simulink model "MPC_point_3"  (R2022a)
settings: Solver=VariableStepAuto  StartTime=0.0  StopTime=T_sim  RelTol=1e-3
values from neighbouring files (symbols this model uses):
  C = [0       1      0  0 ... (first row only)    [main.m]
  C_states = eye(length(A))    [main.m]
  D_states = zeros(length(B), 1)    [main.m]
  N1 = 15    [main.m]
  N2 = 15    [main.m]
  N3 = 100    [main.m]
  N4 = 5    [main.m]
  Q1 = Q_d    [main.m]
  Q2 = Q_d    [main.m]
  Q3 = Q_d    [main.m]
  Q4 = Q_d    [main.m]
  R1 = R_d    (= 10000)    [main.m]
  R2 = R_d    (= 10000)    [main.m]
  R3 = R_d    (= 10000)    [main.m]
  R4 = R_d    (= 10000)    [main.m]
  S1 = Q_d    [main.m]
  S2 = 100 * Q_d    [main.m]
  S3 = Q_d    [main.m]
  S4 = P_d    [main.m]
  sysd = c2d(sys,T_sampling)    [main.m]
  T_sampling = 2*pi/omega_sampling    [main.m]
  u_max = deg2rad(15)    [main.m]
  u_min = deg2rad(-15)    [main.m]
  x0 = [deg2rad(0) deg2rad(15) 0 -300]    [main.m]
  x_ref = [0 0 0 0]    [main.m]
undefined symbols (not defined in the file or in its folder): Klqr_d, mpc_point_3
settings Model: Creator=PaoloA  LastModifiedBy=g_mor
settings DebuggingCC: UnconnectedInputMsg=warning  UnconnectedOutputMsg=warning  UnconnectedLineMsg=warning
settings RTWCC: DLArmComputeVersion=19.05

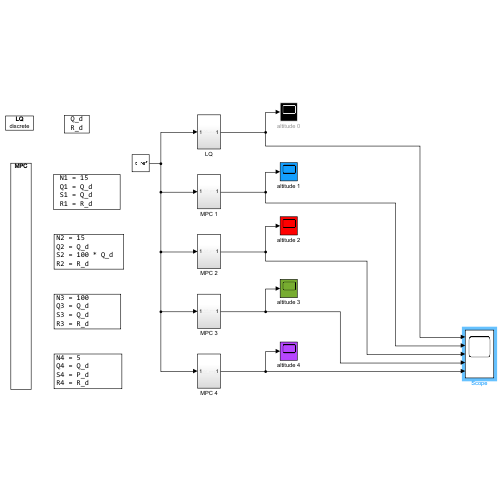
[thumbnail: Simulink's stored preview of the top-level diagram]
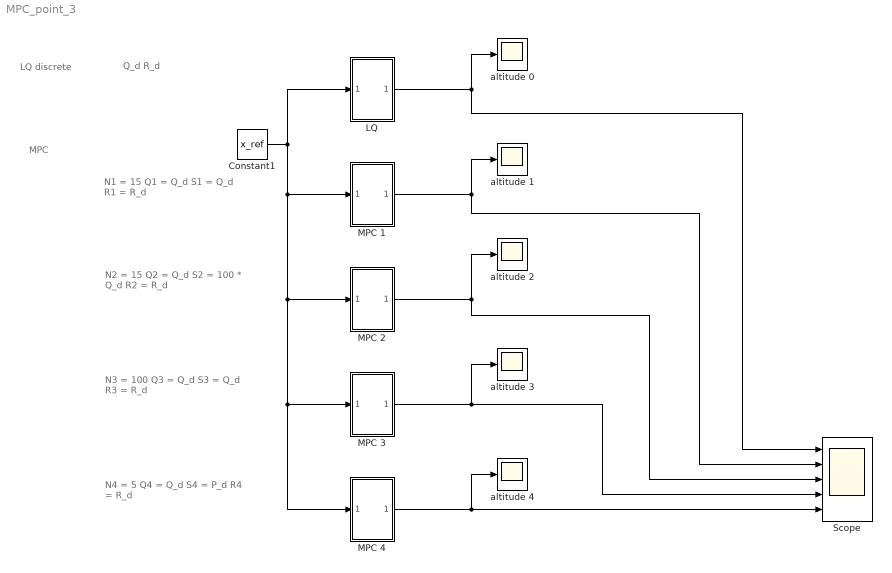
== system MPC_point_3 ==
  note: N4 = 5
      | Q4 = Q_d
      | S4 = P_d
      | R4 = R_d
  note: N3 = 100
      | Q3 = Q_d
      | S3 = Q_d
      | R3 = R_d
  note: N2 = 15
      | Q2 = Q_d
      | S2 = 100 * Q_d
      | R2 = R_d
  note: N1 = 15
      | Q1 = Q_d
      | S1 = Q_d
      | R1 = R_d
  note: MPC
  note: LQ
      | discrete
  note: Q_d
      | R_d
  Constant1 : Constant  Value=x_ref
  LQ : Subsystem
  MPC 1 : Subsystem
  MPC 2 : Subsystem
  MPC 3 : Subsystem
  MPC 4 : Subsystem
  Scope : Scope  NumInputPorts=5
  altitude {0..4} (5 alike) : Scope
  wires:
  Constant1/1 -> LQ/1(In1), MPC 4/1(In1), MPC 3/1(In1), MPC 2/1(In1), MPC 1/1(In1)
  LQ/1(Out1) -> Scope/1, altitude 0/1
  MPC 1/1(Out1) -> Scope/2, altitude 1/1
  MPC 2/1(Out1) -> Scope/3, altitude 2/1
  MPC 3/1(Out1) -> Scope/4, altitude 3/1
  MPC 4/1(Out1) -> altitude 4/1, Scope/5

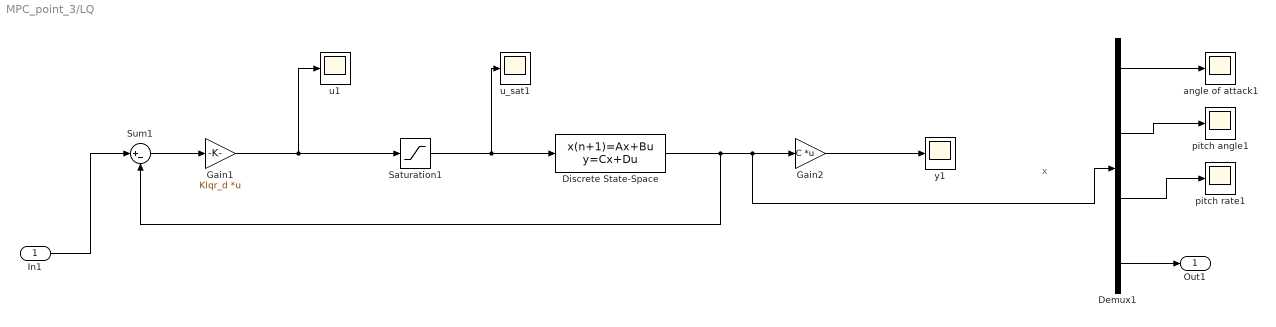
== system MPC_point_3/LQ ==
  note: x
  In1 : Inport
  Demux1 : Demux
  Discrete State-Space : DiscreteStateSpace  A=sysd.A  B=sysd.B  C=C_states  D=D_states  InitialCondition=x0  SampleTime=T_sampling
  Gain1 : Gain  Gain=Klqr_d  Multiplication=Matrix(K*u)
  Gain2 : Gain  Gain=C  Multiplication=Matrix(K*u)
  Saturation1 : Saturate  UpperLimit=u_max  LowerLimit=u_min
  Sum1 : Sum  Inputs=|+-
  angle of attack1 : Scope
  pitch angle1 : Scope
  pitch rate1 : Scope
  u1 : Scope
  u_sat1 : Scope
  y1 : Scope
  Out1 : Outport
  wires:
  Gain2/1 -> y1/1
  Discrete State-Space/1 -> Demux1/1, Gain2/1, Sum1/2
  Saturation1/1 -> Discrete State-Space/1, u_sat1/1
  Gain1/1 -> u1/1, Saturation1/1
  Demux1/4 -> Out1/1
  Demux1/1 -> angle of attack1/1
  Sum1/1 -> Gain1/1
  Demux1/2 -> pitch angle1/1
  Demux1/3 -> pitch rate1/1
  In1/1 -> Sum1/1

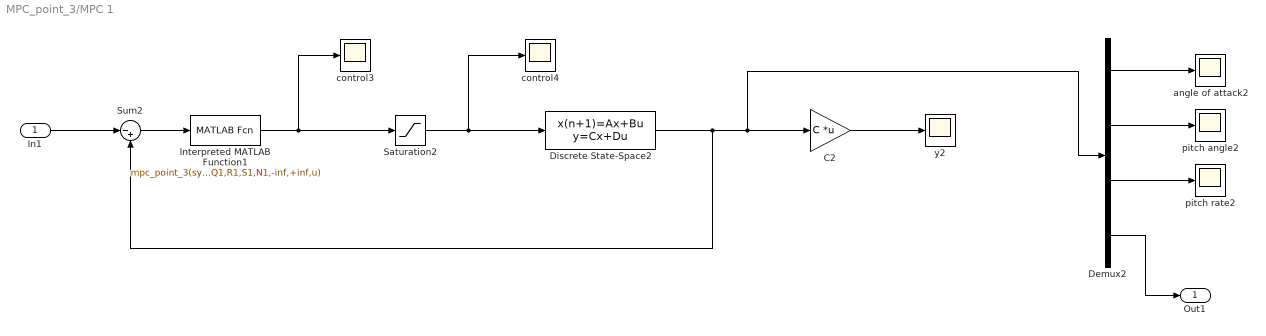
== system MPC_point_3/MPC 1 ==
  In1 : Inport
  C2 : Gain  Gain=C  Multiplication=Matrix(K*u)
  Demux2 : Demux
  Discrete State-Space2 : DiscreteStateSpace  A=sysd.A  B=sysd.B  C=C_states  D=D_states  InitialCondition=x0  SampleTime=T_sampling
  Interpreted MATLAB Function1 : MATLABFcn  MATLABFcn=mpc_point_3(sysd.A,sysd.B,Q1,R1,S1,N1,-inf,+inf,u)  OutputDimensions=1
  Saturation2 : Saturate  UpperLimit=u_max  LowerLimit=u_min
  Sum2 : Sum  Inputs=|-+
  angle of attack2 : Scope
  control3 : Scope
  control4 : Scope
  pitch angle2 : Scope
  pitch rate2 : Scope
  y2 : Scope
  Out1 : Outport
  wires:
  Discrete State-Space2/1 -> C2/1, Demux2/1, Sum2/2
  Saturation2/1 -> Discrete State-Space2/1, control4/1
  In1/1 -> Sum2/1
  Interpreted MATLAB Function1/1 -> Saturation2/1, control3/1
  Sum2/1 -> Interpreted MATLAB Function1/1
  Demux2/2 -> pitch angle2/1
  Demux2/3 -> pitch rate2/1
  C2/1 -> y2/1
  Demux2/1 -> angle of attack2/1
  Demux2/4 -> Out1/1

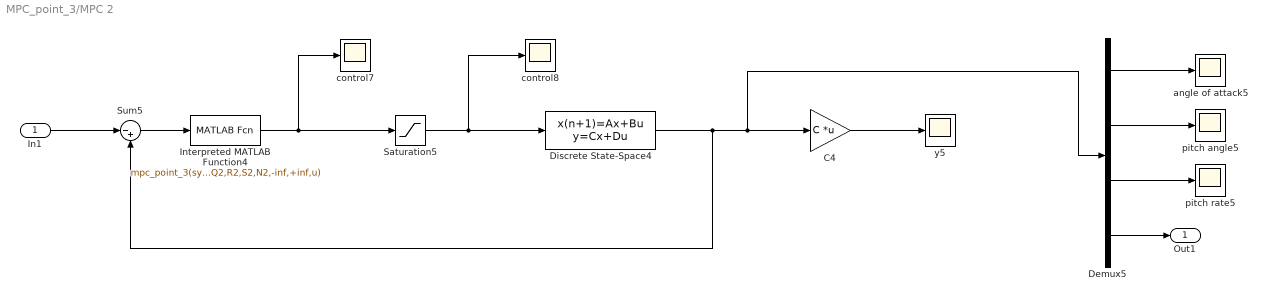
== system MPC_point_3/MPC 2 ==
  In1 : Inport
  C4 : Gain  Gain=C  Multiplication=Matrix(K*u)
  Demux5 : Demux
  Discrete State-Space4 : DiscreteStateSpace  A=sysd.A  B=sysd.B  C=C_states  D=D_states  InitialCondition=x0  SampleTime=T_sampling
  Interpreted MATLAB Function4 : MATLABFcn  MATLABFcn=mpc_point_3(sysd.A,sysd.B,Q2,R2,S2,N2,-inf,+inf,u)  OutputDimensions=1
  Saturation5 : Saturate  UpperLimit=u_max  LowerLimit=u_min
  Sum5 : Sum  Inputs=|-+
  angle of attack5 : Scope
  control7 : Scope
  control8 : Scope
  pitch angle5 : Scope
  pitch rate5 : Scope
  y5 : Scope
  Out1 : Outport
  wires:
  Saturation5/1 -> Discrete State-Space4/1, control8/1
  Discrete State-Space4/1 -> C4/1, Demux5/1, Sum5/2
  Interpreted MATLAB Function4/1 -> Saturation5/1, control7/1
  C4/1 -> y5/1
  Sum5/1 -> Interpreted MATLAB Function4/1
  Demux5/2 -> pitch angle5/1
  Demux5/3 -> pitch rate5/1
  Demux5/1 -> angle of attack5/1
  In1/1 -> Sum5/1
  Demux5/4 -> Out1/1

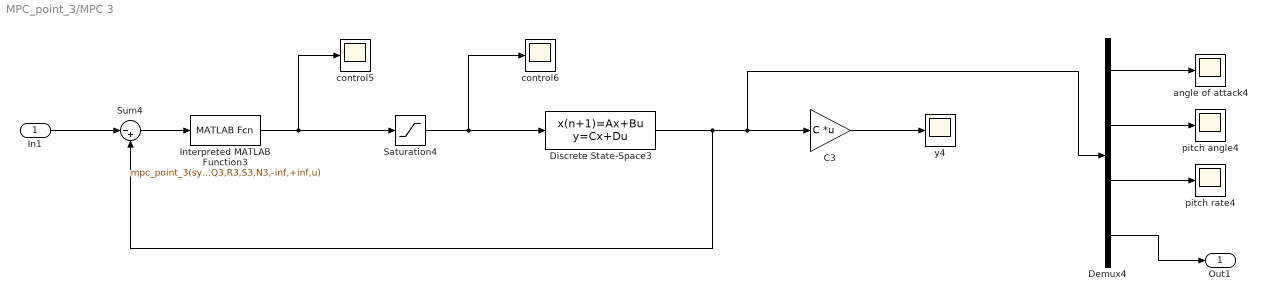
== system MPC_point_3/MPC 3 ==
  In1 : Inport
  C3 : Gain  Gain=C  Multiplication=Matrix(K*u)
  Demux4 : Demux
  Discrete State-Space3 : DiscreteStateSpace  A=sysd.A  B=sysd.B  C=C_states  D=D_states  InitialCondition=x0  SampleTime=T_sampling
  Interpreted MATLAB Function3 : MATLABFcn  MATLABFcn=mpc_point_3(sysd.A,sysd.B,Q3,R3,S3,N3,-inf,+inf,u)  OutputDimensions=1
  Saturation4 : Saturate  UpperLimit=u_max  LowerLimit=u_min
  Sum4 : Sum  Inputs=|-+
  angle of attack4 : Scope
  control5 : Scope
  control6 : Scope
  pitch angle4 : Scope
  pitch rate4 : Scope
  y4 : Scope
  Out1 : Outport
  wires:
  Discrete State-Space3/1 -> C3/1, Demux4/1, Sum4/2
  Demux4/1 -> angle of attack4/1
  Demux4/3 -> pitch rate4/1
  C3/1 -> y4/1
  Demux4/2 -> pitch angle4/1
  Interpreted MATLAB Function3/1 -> Saturation4/1, control5/1
  Saturation4/1 -> Discrete State-Space3/1, control6/1
  Sum4/1 -> Interpreted MATLAB Function3/1
  In1/1 -> Sum4/1
  Demux4/4 -> Out1/1

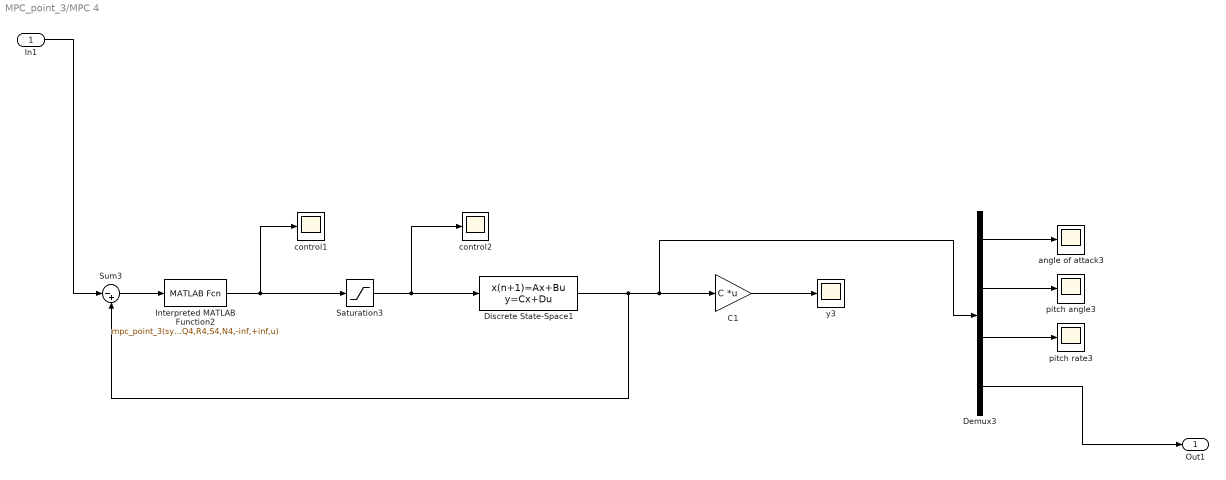
== system MPC_point_3/MPC 4 ==
  In1 : Inport
  C1 : Gain  Gain=C  Multiplication=Matrix(K*u)
  Demux3 : Demux
  Discrete State-Space1 : DiscreteStateSpace  A=sysd.A  B=sysd.B  C=C_states  D=D_states  InitialCondition=x0  SampleTime=T_sampling
  Interpreted MATLAB Function2 : MATLABFcn  MATLABFcn=mpc_point_3(sysd.A,sysd.B,Q4,R4,S4,N4,-inf,+inf,u)  OutputDimensions=1
  Saturation3 : Saturate  UpperLimit=u_max  LowerLimit=u_min
  Sum3 : Sum  Inputs=|-+
  angle of attack3 : Scope
  control1 : Scope
  control2 : Scope
  pitch angle3 : Scope
  pitch rate3 : Scope
  y3 : Scope
  Out1 : Outport
  wires:
  Demux3/1 -> angle of attack3/1
  Saturation3/1 -> Discrete State-Space1/1, control2/1
  Demux3/3 -> pitch rate3/1
  Discrete State-Space1/1 -> C1/1, Demux3/1, Sum3/2
  Demux3/2 -> pitch angle3/1
  C1/1 -> y3/1
  Interpreted MATLAB Function2/1 -> Saturation3/1, control1/1
  Sum3/1 -> Interpreted MATLAB Function2/1
  Demux3/4 -> Out1/1
  In1/1 -> Sum3/1
